simulink model "lab_10_target"  (R2023b)
settings: Solver=VariableStepAuto  StartTime=0.0  StopTime=10.0  RelTol=1e-3
libraries: speedgoatlib_IO102 x2

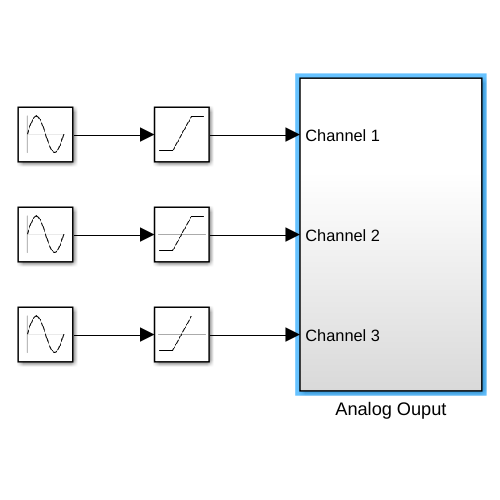
[thumbnail: Simulink's stored preview of the top-level diagram]
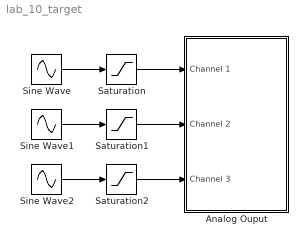
== system lab_10_target ==
  Analog Ouput : Subsystem
  Saturation : Saturate
  Saturation1 : Saturate
  Saturation2 : Saturate
  Sine Wave : Sin  Amplitude=0.5  Frequency=5*pi/180  SampleTime=0
  Sine Wave1 : Sin  Amplitude=0.5  Frequency=5*pi/180  Phase=2/3*pi  SampleTime=0
  Sine Wave2 : Sin  Amplitude=0.5  Frequency=5*pi/180  Phase=-2/3*pi  SampleTime=0
  wires:
  Sine Wave/1 -> Saturation/1
  Saturation/1 -> Analog Ouput/1(Channel 1)
  Sine Wave1/1 -> Saturation1/1
  Saturation1/1 -> Analog Ouput/2(Channel 2)
  Sine Wave2/1 -> Saturation2/1
  Saturation2/1 -> Analog Ouput/3(Channel 3)

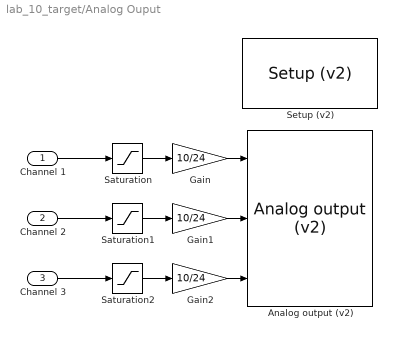
== system lab_10_target/Analog Ouput ==
  Channel 1 : Inport
  Channel 2 : Inport  Port=2
  Channel 3 : Inport  Port=3
  "Analog output (v2) " : speedgoatlib_IO102/Analog output (v2)   id=1  channels=[1 2 3]  range=1  ts=-1  pciSlot=-1
  Gain : Gain  Gain=10/24
  Gain1 : Gain  Gain=10/24
  Gain2 : Gain  Gain=10/24
  Saturation : Saturate  UpperLimit=24  LowerLimit=-24
  Saturation1 : Saturate  UpperLimit=24  LowerLimit=-24
  Saturation2 : Saturate  UpperLimit=24  LowerLimit=-24
  "Setup (v2) " : speedgoatlib_IO102/Setup (v2)   id=1  range=+-10V  cal=off  pciSlot=-1  adCoupling=Single-ended  adChannelMode=Multiple-channel (enter number of channels below)  adChannel=4  daChannel=[1,2,3]  daInitValue=[0]  daReset=[1]  DioDirectionLo=Input  DioDirectionHi=Output  doChannel=[9]  doInitValue=[0]  doReset=[1]  diChannel=[1]
  wires:
  Saturation/1 -> Gain/1
  Saturation1/1 -> Gain1/1
  Saturation2/1 -> Gain2/1
  Gain1/1 -> "Analog output (v2) "/2
  Gain/1 -> "Analog output (v2) "/1
  Gain2/1 -> "Analog output (v2) "/3
  Channel 2/1 -> Saturation1/1
  Channel 3/1 -> Saturation2/1
  Channel 1/1 -> Saturation/1
